simulink model "Throttle_Position_Sensors"  (R2023a)
settings: Solver=VariableStepAuto  StartTime=0.0  StopTime=10  RelTol=1e-3
settings Model: Creator=ItShop  LastModifiedBy=ItShop

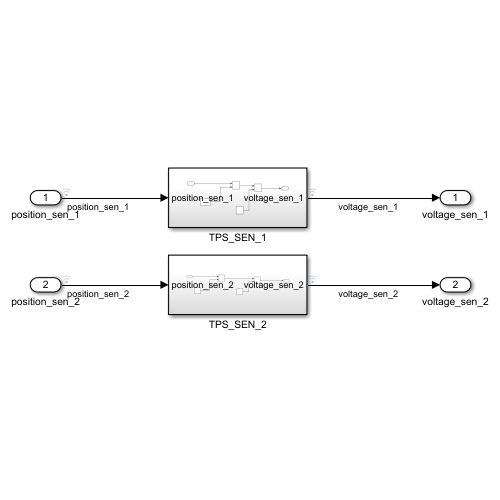
[thumbnail: Simulink's stored preview of the top-level diagram]
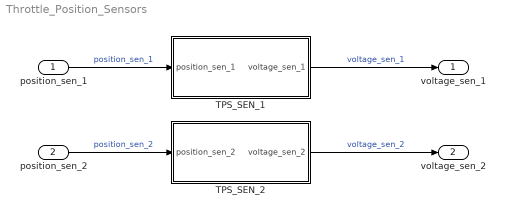
== system Throttle_Position_Sensors ==
  position_sen_1 : Inport
  position_sen_2 : Inport  Port=2
  TPS_SEN_1 : Subsystem
  TPS_SEN_2 : Subsystem
  voltage_sen_1 : Outport
  voltage_sen_2 : Outport  Port=2
  wires:
  position_sen_1/1 -> TPS_SEN_1/1(position_sen_1)  "position_sen_1"
  TPS_SEN_1/1(voltage_sen_1) -> voltage_sen_1/1  "voltage_sen_1"
  position_sen_2/1 -> TPS_SEN_2/1(position_sen_2)  "position_sen_2"
  TPS_SEN_2/1(voltage_sen_2) -> voltage_sen_2/1  "voltage_sen_2"

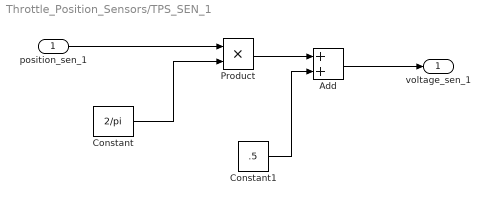
== system Throttle_Position_Sensors/TPS_SEN_1 ==
  position_sen_1 : Inport
  Add : Sum
  Constant : Constant  Value=2/pi
  Constant1 : Constant  Value=.5
  Product : Product
  voltage_sen_1 : Outport
  wires:
  position_sen_1/1 -> Product/1
  Constant/1 -> Product/2
  Constant1/1 -> Add/2
  Product/1 -> Add/1
  Add/1 -> voltage_sen_1/1

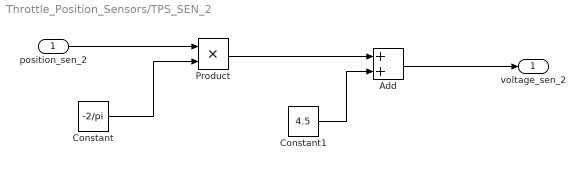
== system Throttle_Position_Sensors/TPS_SEN_2 ==
  position_sen_2 : Inport
  Add : Sum
  Constant : Constant  Value=-2/pi
  Constant1 : Constant  Value=4.5
  Product : Product
  voltage_sen_2 : Outport
  wires:
  position_sen_2/1 -> Product/1
  Constant/1 -> Product/2
  Constant1/1 -> Add/2
  Product/1 -> Add/1
  Add/1 -> voltage_sen_2/1
